simulink model "StateMachinaTesting"  (R2016a)
settings: Solver=VariableStepAuto  StartTime=0.0  StopTime=orbit_length*40  RelTol=1e-3
values from neighbouring files (symbols this model uses):
  A = eye(16,16)    [full_input_list.m]
  B = zeros(16,1)    [full_input_list.m]
  C = blkdiag(eye(3,3),zeros(3,3),eye(10,10))    [full_input_list.m]
  counter = 0    [full_input_list.m]
  deltaT = 0.00001    (= 1e-05)    [full_input_list.m]
  H = C    [full_input_list.m]
  kd = 0.5    [full_input_list.m]    (also in initACS.m = 0.01)
  kp = 1    [full_input_list.m]    (also in initACS.m = 0.01)
  OpModes = [0 0 0]    [full_input_list.m]
  OpTimes = [0 1 2]    [full_input_list.m]
  Q_k = zeros(16,16)    [full_input_list.m]
  R = R_k    [full_input_list.m]
  SeperationTime = 30000    [full_input_list.m]
  sim_start_time = (JD - JD_GPS0) * 24*60*60 - UTC_leap_seconds_wrt_GPS    (= 36000.0287935)    [full_input_list.m]
  st = 1/freq    (= 0.0125)    [full_input_list.m]    (also in initSimulink.m)
  u_k = zeros(16,1)    [full_input_list.m]
  w_k = zeros(16,1)    [full_input_list.m]
  x0 = [0 ... (first row only)    [full_input_list.m]
  Z_k = zeros(16,1)    [full_input_list.m]
undefined symbols (not defined in the file or in its folder): DiscIntNeverNeededParam, Earth, G_igrf, gyro_DCM_BS, H_igrf, I_undeployed, IAU, km, Kschmidt, mag_variance, n, R_mean, sat2, WGS84
libraries: simulink x29, dspmathops x24, aerolibutil x20, aerolibtransform2 x20, vrlib x15, aerolibgravity2 x5, dspinverses x4, SimMainLibrary x3, dspmtrx3 x1, lib_violet_env x1
(part 1 of 4)
settings Model: Creator=npp26  LastModifiedBy=gtc59

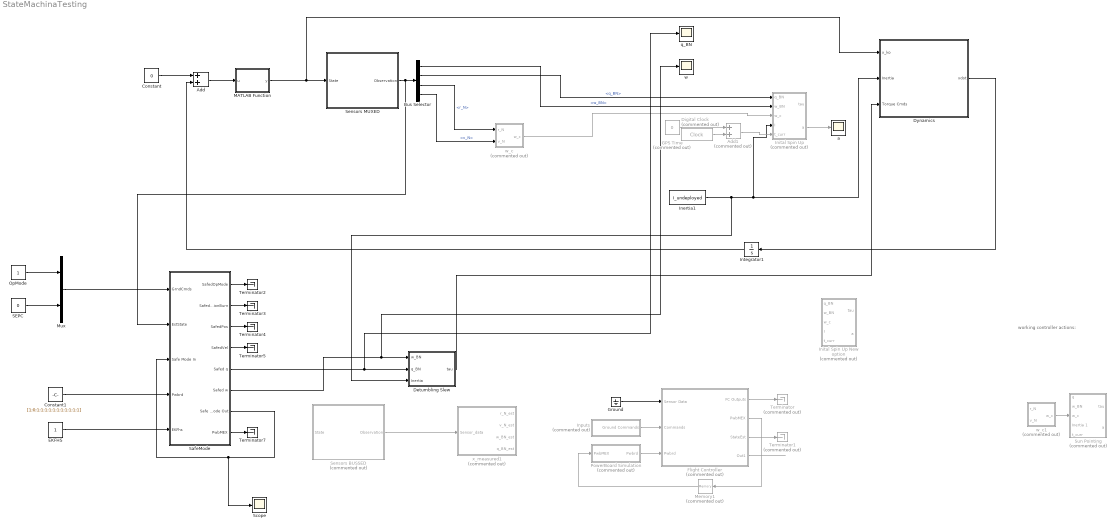
== system StateMachinaTesting ==
  note: working controller actions:
  Add : Sum
  Add1 : Sum  Commented=on
  Bus Selector : BusSelector  OutputSignals=w_BN,q_BN,r_N,v_N
  Constant : Constant  Value=0
  Constant1 : Constant  Value=[1;0;1;1;1;1;1;1;1;1;1;1;1]
  Detumbling Slew : Subsystem  TreatAsAtomicUnit=on
  Digital Clock : DigitalClock  Commented=on
  "Dynamics " : Subsystem
  EKFHS : Constant
  Flight Controller : Subsystem  Commented=on
  GPS Time : Constant  Commented=on  Value=0
  Ground : Ground
  Inertia1 : Constant  Value=I_undeployed
  Inital Spin Up : Subsystem  Commented=on  TreatAsAtomicUnit=on
  Inital Spin Up New option : Subsystem  Commented=on  TreatAsAtomicUnit=on
  Inputs : Subsystem  Commented=on
  Integrator1 : Integrator  InitialCondition=x0
  MATLAB Function : MATLAB Function  TreatAsAtomicUnit=on
  Memory1 : Memory  Commented=on  InheritSampleTime=on
  Mux : Mux  Inputs=2
  OpMode : Constant
  PowerBoard Simulation : Subsystem  Commented=on
  SEPC : Constant  Value=0
  SafeMode : Subsystem
  Scope : Scope
  Sensors BUSSED : Subsystem  Commented=on
  Sensors MUXED : Subsystem
  Sun Pointing : Subsystem  Commented=on  TreatAsAtomicUnit=on
  Terminator : Terminator  Commented=on
  Terminator1 : Terminator  Commented=on
  Terminator{2..5,7} (5 alike) : Terminator
  a : Scope
  q_BN : Scope
  w : Scope
  w_c : Subsystem  Commented=on
  w_c1 : Subsystem  Commented=on
  x_measured1 : Subsystem  Commented=on
  wires:
  "Dynamics "/1("xdot  ") -> Integrator1/1
  Constant/1 -> Add/1
  Integrator1/1 -> Add/2
  Add/1 -> MATLAB Function/1(u)
  Inertia1/1 -> Detumbling Slew/3("Inertia "), Inital Spin Up/4("I "), "Dynamics "/2(Inertia)
  Inputs/1(Ground Commands) -> Flight Controller/2(Commands)
  PowerBoard Simulation/1(Pwbrd) -> Flight Controller/3(Pwbrd)
  Flight Controller/2(PwbMEX) -> Memory1/1
  Memory1/1 -> PowerBoard Simulation/1(PwbMEX)
  Ground/1 -> Flight Controller/1(Sensor Data)
  Flight Controller/1(FC Outputs) -> Terminator/1
  Flight Controller/3(StateEst) -> Terminator1/1
  Flight Controller/4(Out1) -> ?
  Bus Selector/2 -> Inital Spin Up/1(q_BN)  "<q_BN>"
  Bus Selector/1 -> Inital Spin Up/2(w_BN)  "<w_BN>"
  Sensors BUSSED/1(Observation) -> x_measured1/1(Sensor_data)
  Sensors MUXED/1(Observation) -> SafeMode/2(EstState), Bus Selector/1
  MATLAB Function/1(y) -> Sensors MUXED/1(State), "Dynamics "/1("x_ko ")
  Bus Selector/3 -> w_c/1(r_N)  "<r_N>"
  Bus Selector/4 -> w_c/2(v_N)  "<v_N>"
  w_c/1(w_c) -> Inital Spin Up/3(w_c)
  Inital Spin Up/2(a) -> a/1
  w_c1/1(w_c) -> Sun Pointing/3(w_c)
  GPS Time/1 -> Add1/1
  Digital Clock/1 -> Add1/2
  Add1/1 -> Inital Spin Up/5(t_curr)
  SafeMode/5(Safed q) -> q_BN/1, Detumbling Slew/2(q_BN)
  SafeMode/6(Safed w) -> w/1, Detumbling Slew/1(w_BN)
  SafeMode/1(SafedOpMode) -> Terminator2/1
  SafeMode/2(SafedSeperationBurn) -> Terminator3/1
  SafeMode/3(SafedPos) -> Terminator4/1
  SafeMode/4(SafedVel) -> Terminator5/1
  SafeMode/7(Safe Mode Out) -> Scope/1, SafeMode/3(Safe Mode In)
  SafeMode/8(PwbMEX) -> Terminator7/1
  OpMode/1 -> Mux/1
  SEPC/1 -> Mux/2
  Mux/1 -> SafeMode/1(GrndCmds)
  Constant1/1 -> SafeMode/4(Pwbrd)
  EKFHS/1 -> SafeMode/5("EKFhs ")
  Detumbling Slew/1(tau) -> "Dynamics "/3(Torque Cmds)

== system StateMachinaTesting/Detumbling Slew ==
  note: Regulator
      | - q_target = [0 0 0 1]
      | - w_target = [0 0 0]
  note: Markley Regulator
      | This regulator takes the current directional quaterion vector, the target quaterion, the intertial matrix, and the current angular velocity to determine the required torque necessary to the slew.
      |
      | The equation is 7.8 listed on page 290 of Fundamentals of Spacecraft Attitude Determination and Control. The input I is currently not defined. Also important to the equation is equation 7.2
  w_BN : Inport
  q_BN : Inport  Port=2
  "Inertia " : Inport  Port=3
  3x3 Cross Product : aerolibutil/3x3 Cross Product
  Add : Sum  Inputs=+++
  Constant : Constant  Commented=on  Value=[0;0;0]
  Gain : Gain  Gain=-1
  Gain1 : Gain  Gain=kp
  Gain2 : Gain  Gain=-1
  Gain3 : Gain  Gain=kd
  Gain4 : Gain  Gain=-1
  Product : Product  Multiplication=Matrix(*)
  Quaternion Inverse : aerolibutil/Quaternion Inverse
  Quaternion Multiplication : aerolibutil/Quaternion Multiplication
  Selector : Selector  InputPortWidth=4  IndexOptions=Index vector (dialog)  Indices=[1 2 3]  OutputSizes=1
  Target q : Constant  Value=[ 0 0 0 1 ]
  tau : Outport
  wires:
  Target q/1 -> Quaternion Inverse/1
  Quaternion Multiplication/1 -> Selector/1
  Selector/1 -> Gain1/1
  Gain1/1 -> Gain/1
  Gain3/1 -> Gain2/1
  w_BN/1 -> 3x3 Cross Product/1, Gain3/1, Product/2
  Gain/1 -> Add/1
  Gain2/1 -> Add/2
  "Inertia "/1 -> Product/1
  Product/1 -> 3x3 Cross Product/2
  3x3 Cross Product/1 -> Gain4/1
  Gain4/1 -> Add/3
  Add/1 -> tau/1
  Quaternion Inverse/1 -> Quaternion Multiplication/1
  q_BN/1 -> Quaternion Multiplication/2

== system StateMachinaTesting/Dynamics  ==
  note: State x {16x1} =
      | x y z - Position
      | xdot ydot zdot - Velocity
      | xddot yddot zddot - Accel
      | w1 w2 w3 - Angular Vel
      | q1 q2 q3 q4 - Quaternion
  "x_ko " : Inport
  Inertia : Inport  Port=2
  Torque Cmds : Inport  Port=3
  Dynamics of the System : MATLAB Function  TreatAsAtomicUnit=on
  "xdot  " : Outport
  wires:
  Dynamics of the System/1(xdot) -> "xdot  "/1
  Torque Cmds/1 -> Dynamics of the System/3(torques)
  Inertia/1 -> Dynamics of the System/2(Inertia)
  "x_ko "/1 -> Dynamics of the System/1(x_ko)

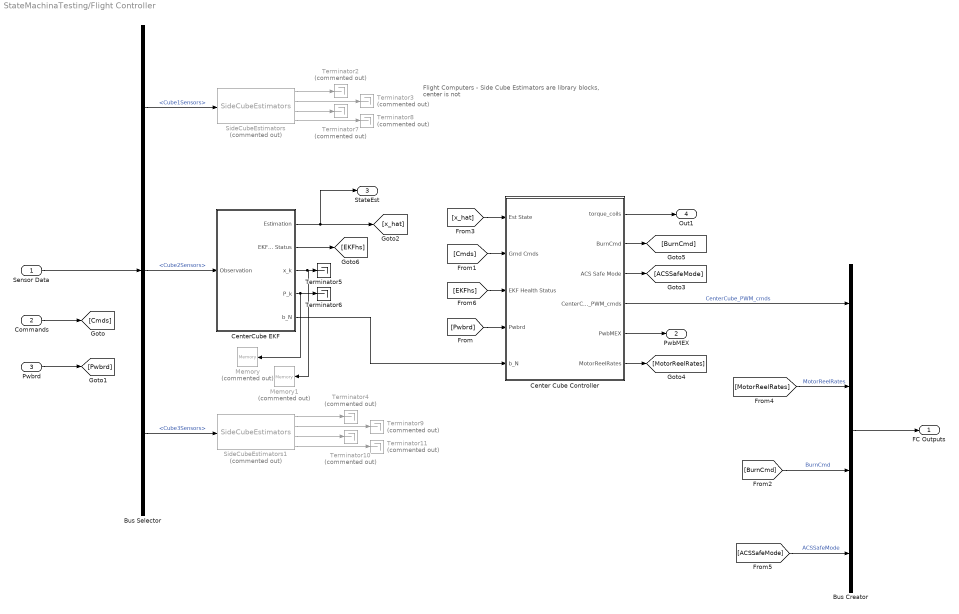
== system StateMachinaTesting/Flight Controller ==
  note: Flight Computers
      | - Side Cube Estimators are library blocks, center is not
  Sensor Data : Inport
  Commands : Inport  Port=2
  Pwbrd : Inport  Port=3
  Bus Creator : BusCreator  Inputs=4
  Bus Selector : BusSelector  OutputSignals=Cube1Sensors,Cube2Sensors,Cube3Sensors
  Center Cube Controller : Subsystem
  CenterCube EKF : Subsystem
  Memory : Memory  Commented=on
  Memory1 : Memory  Commented=on
  SideCubeEstimators : SimMainLibrary/SideCubeEstimators  Commented=on
  SideCubeEstimators1 : SimMainLibrary/SideCubeEstimators  Commented=on
  Terminator{2..4,7..11} (8 alike) : Terminator  Commented=on
  Terminator5 : Terminator
  Terminator6 : Terminator
  FC Outputs : Outport
  PwbMEX : Outport  Port=2
  StateEst : Outport  Port=3
  Out1 : Outport  Port=4
  wires:
  Sensor Data/1 -> Bus Selector/1
  Bus Selector/1 -> SideCubeEstimators/1  "<Cube1Sensors>"
  Bus Selector/2 -> CenterCube EKF/1(Observation)  "<Cube2Sensors>"
  Bus Selector/3 -> SideCubeEstimators1/1  "<Cube3Sensors>"
  SideCubeEstimators/1 -> Terminator2/1
  Bus Creator/1 -> FC Outputs/1
  Commands/1 -> [Cmds]
  [Cmds] -> Center Cube Controller/2(Grnd Cmds)
  Center Cube Controller/3(ACS Safe Mode) -> [ACSSafeMode]
  Center Cube Controller/2(BurnCmd) -> [BurnCmd]
  [BurnCmd] -> Bus Creator/3  "BurnCmd"
  CenterCube EKF/2(EKF Health Status) -> [EKFhs]
  [EKFhs] -> Center Cube Controller/3("EKF Health Status ")
  Pwbrd/1 -> [Pwbrd]
  [Pwbrd] -> Center Cube Controller/4(Pwbrd)
  Center Cube Controller/5(PwbMEX) -> PwbMEX/1
  CenterCube EKF/1(Estimation) -> [x_hat], StateEst/1
  [x_hat] -> Center Cube Controller/1(Est State)
  Center Cube Controller/4(CenterCube_PWM_cmds) -> Bus Creator/1  "CenterCube_PWM_cmds"
  SideCubeEstimators/2 -> Terminator3/1
  CenterCube EKF/3(x_k) -> Memory1/1, Terminator5/1
  CenterCube EKF/4(P_k) -> Terminator6/1, Memory/1
  SideCubeEstimators/3 -> Terminator7/1
  SideCubeEstimators/4 -> Terminator8/1
  SideCubeEstimators1/1 -> Terminator4/1
  SideCubeEstimators1/2 -> Terminator9/1
  SideCubeEstimators1/3 -> Terminator10/1
  SideCubeEstimators1/4 -> Terminator11/1
  [ACSSafeMode] -> Bus Creator/4  "ACSSafeMode"
  Center Cube Controller/6(MotorReelRates) -> [MotorReelRates]
  [MotorReelRates] -> Bus Creator/2  "MotorReelRates"
  Center Cube Controller/1(torque_coils) -> Out1/1
  CenterCube EKF/5(b_N) -> Center Cube Controller/5(b_N)

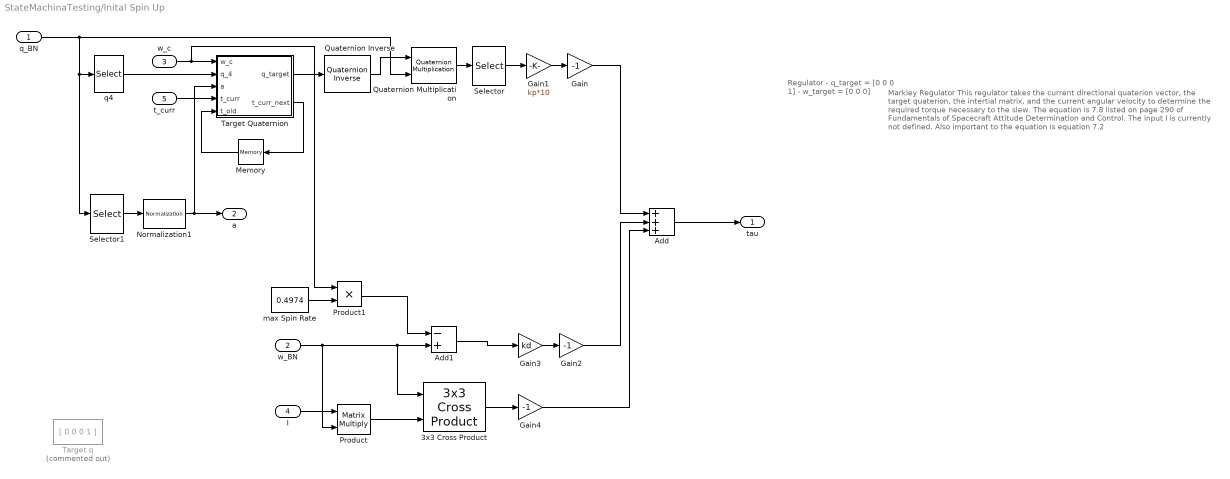
== system StateMachinaTesting/Inital Spin Up ==
  note: Regulator
      | - q_target = [0 0 0 1]
      | - w_target = [0 0 0]
  note: Markley Regulator
      | This regulator takes the current directional quaterion vector, the target quaterion, the intertial matrix, and the current angular velocity to determine the required torque necessary to the slew.
      |
      | The equation is 7.8 listed on page 290 of Fundamentals of Spacecraft Attitude Determination and Control. The input I is currently not defined. Also important to the equation is equation 7.2
  q_BN : Inport
  w_BN : Inport  Port=2
  w_c : Inport  Port=3
  "I " : Inport  Port=4
  t_curr : Inport  Port=5
  3x3 Cross Product : aerolibutil/3x3 Cross Product
  Add : Sum  Inputs=+++
  Add1 : Sum  Inputs=-+
  Gain : Gain  Gain=-1
  Gain1 : Gain  Gain=kp*10
  Gain2 : Gain  Gain=-1
  Gain3 : Gain  Gain=kd
  Gain4 : Gain  Gain=-1
  Memory : Memory
  Normalization1 : dspmathops/Normalization  NormType=2-norm  Bias=1e-10  NormOver=Each column  Dimension=1  outputDataTypeStr=Inherit: Same as product output  outputLastDataTypeStr=Inherit: Same as product output  outputMin=[]  outputMax=[]  accumDataTypeStr=Inherit: Same as product output  accumLastDataTypeStr=Inherit: Same as product output  roundingMode=Floor  overflowMode=off
  Product : Product  Multiplication=Matrix(*)
  Product1 : Product
  Quaternion Inverse : aerolibutil/Quaternion Inverse
  Quaternion Multiplication : aerolibutil/Quaternion Multiplication
  Selector : Selector  InputPortWidth=4  IndexOptions=Index vector (dialog)  Indices=[1 2 3]  OutputSizes=1
  Selector1 : Selector  InputPortWidth=4  IndexOptions=Index vector (dialog)  Indices=[1 2 3]  OutputSizes=1
  Target Quaternion : Subsystem
  Target q : Constant  Commented=on  Value=[ 0 0 0 1 ]
  max Spin Rate : Constant  Value=0.4974
  q4 : Selector  InputPortWidth=4  IndexOptions=Index vector (dialog)  Indices=[4]  OutputSizes=1
  tau : Outport
  a : Outport  Port=2
  wires:
  Target Quaternion/1(q_target) -> Quaternion Inverse/1
  Quaternion Multiplication/1 -> Selector/1
  Selector/1 -> Gain1/1
  Gain1/1 -> Gain/1
  Gain3/1 -> Gain2/1
  w_BN/1 -> Product/2, Add1/2, 3x3 Cross Product/1
  Add/1 -> tau/1
  Gain/1 -> Add/1
  Gain2/1 -> Add/2
  "I "/1 -> Product/1
  Product/1 -> 3x3 Cross Product/2
  3x3 Cross Product/1 -> Gain4/1
  Gain4/1 -> Add/3
  w_c/1 -> Product1/1, Target Quaternion/1(w_c)
  Selector1/1 -> Normalization1/1
  Normalization1/1 -> a/1, Target Quaternion/3(a)
  t_curr/1 -> Target Quaternion/4(t_curr)
  q4/1 -> Target Quaternion/2(q_4)
  Target Quaternion/2(t_curr_next) -> Memory/1
  Memory/1 -> Target Quaternion/5(t_old)
  q_BN/1 -> Quaternion Multiplication/2, Selector1/1, q4/1
  max Spin Rate/1 -> Product1/2
  Add1/1 -> Gain3/1
  Product1/1 -> Add1/1
  Quaternion Inverse/1 -> Quaternion Multiplication/1

== system StateMachinaTesting/Inital Spin Up New option ==
  note: Markley Regulator
      | This regulator takes the current directional quaterion vector, the target quaterion, the intertial matrix, and the current angular velocity to determine the required torque necessary to the slew.
      |
      | The equation is 7.8 listed on page 290 of Fundamentals of Spacecraft Attitude Determination and Control. The input I is currently not defined. Also important to the equation is equation 7.2
  note: Regulator
      | - q_target = [0 0 0 1]
      | - w_target = [0 0 0]
  q_BN : Inport
  w_BN : Inport  Port=2
  w_c : Inport  Port=3
  "I " : Inport  Port=4
  t_curr : Inport  Port=5
  3x3 Cross Product : aerolibutil/3x3 Cross Product
  Add : Sum  Inputs=+++
  Add1 : Sum  Inputs=-+
  Add2 : Sum  Inputs=-+
  Gain : Gain  Gain=-1
  Gain1 : Gain  Gain=kp
  Gain2 : Gain  Gain=-1
  Gain3 : Gain  Gain=kd
  Gain4 : Gain  Gain=-1
  Normalization1 : dspmathops/Normalization  NormType=2-norm  Bias=1e-10  NormOver=Each column  Dimension=1  outputDataTypeStr=Inherit: Same as product output  outputLastDataTypeStr=Inherit: Same as product output  outputMin=[]  outputMax=[]  accumDataTypeStr=Inherit: Same as product output  accumLastDataTypeStr=Inherit: Same as product output  roundingMode=Floor  overflowMode=off
  Product : Product  Multiplication=Matrix(*)
  Product1 : Product
  Selector1 : Selector  InputPortWidth=4  IndexOptions=Index vector (dialog)  Indices=[1 2 3]  OutputSizes=1
  Terminator : Terminator
  max Spin Rate : Constant  Value=0.4974
  tau : Outport
  a : Outport  Port=2
  wires:
  Normalization1/1 -> a/1
  Selector1/1 -> Normalization1/1
  Gain4/1 -> Add/3
  3x3 Cross Product/1 -> Gain4/1
  Product/1 -> Add1/1, 3x3 Cross Product/2
  "I "/1 -> Product/1
  Gain2/1 -> Add/2
  Gain/1 -> Add/1
  Add/1 -> tau/1
  w_BN/1 -> 3x3 Cross Product/1, Add2/2, Product/2
  Gain3/1 -> Gain2/1
  Gain1/1 -> Gain/1
  Add1/1 -> Gain1/1
  q_BN/1 -> Selector1/1
  t_curr/1 -> Terminator/1
  w_c/1 -> Add1/2, Product1/1
  max Spin Rate/1 -> Product1/2
  Product1/1 -> Add2/1
  Add2/1 -> Gain3/1

== system StateMachinaTesting/Inputs ==
  Bus Creator : BusCreator  Inputs=2
  Choose Mode : MATLAB Function  TreatAsAtomicUnit=on
  Clock : Clock
  Constant : Constant  Value=OpModes
  Constant1 : Constant  Value=OpTimes
  Constant2 : Constant  Value=SeperationTime
  Ground Commands : Outport
  wires:
  Constant/1 -> Choose Mode/3(OpModes)
  Constant1/1 -> Choose Mode/2(OpTimes)
  Clock/1 -> Choose Mode/1(time)
  Constant2/1 -> Choose Mode/4(SeperationTime)
  Choose Mode/1(OM) -> Bus Creator/1  "OpMode"
  Choose Mode/2(SEPC) -> Bus Creator/2  "SeperationCommand"
  Bus Creator/1 -> Ground Commands/1

== system StateMachinaTesting/PowerBoard Simulation ==
  PwbMEX : Inport
  Bus Creator : BusCreator  Inputs=2
  Bus Creator1 : BusCreator  Inputs=8
  Bus Creator2 : BusCreator  Inputs=3
  Bus Creator3 : BusCreator  Inputs=2
  Bus Creator4 : BusCreator  Inputs=2
  Choose Mode : MATLAB Function  TreatAsAtomicUnit=on
  Clock : Clock
  Constant : Constant  Value=OpModes
  Constant1 : Constant  Value=OpTimes
  Constant2 : Constant  Value=SeperationTime
  Sensor Ak Signals : Subsystem
  Torquer Shunts : Subsystem
  Pwbrd : Outport
  wires:
  Constant/1 -> Choose Mode/4(OpModes)
  Constant1/1 -> Choose Mode/3(OpTimes)
  Clock/1 -> Choose Mode/2(time)
  Constant2/1 -> Choose Mode/5(SeperationTime)
  Choose Mode/1(OM) -> Bus Creator/1  "PbOpMode"
  Choose Mode/2(SEPC) -> Bus Creator/2  "PbSepCmmd"
  Bus Creator/1 -> Bus Creator4/1  "PwbrdCmmds"
  Sensor Ak Signals/4(Out4) -> Bus Creator1/4  "Accel2Ak"
  Sensor Ak Signals/3(Out3) -> Bus Creator1/3  "Accel1Ak"
  Sensor Ak Signals/1(Out1) -> Bus Creator1/1  "Mag1Ak"
  Sensor Ak Signals/2(Out2) -> Bus Creator1/2  "Mag2Ak"
  Bus Creator1/1 -> Bus Creator3/1  "SensorsAk"
  Torquer Shunts/1(Torquer X1 Shunt) -> Bus Creator2/1  "TC_X1"
  Torquer Shunts/2(Torquer Y1 Shunt) -> Bus Creator2/2  "TC_Y1"
  Torquer Shunts/3(Torquer Z1 Shunt) -> Bus Creator2/3  "TC_Z1"
  Bus Creator2/1 -> Bus Creator3/2  "TorquerAk"
  Bus Creator3/1 -> Bus Creator4/2  "ADCSAks"
  Bus Creator4/1 -> Pwbrd/1
  Sensor Ak Signals/5(Out5) -> Bus Creator1/5  "Gyro1Ak"
  Sensor Ak Signals/6(Out6) -> Bus Creator1/6  "Gyro2Ak"
  Sensor Ak Signals/7(Out7) -> Bus Creator1/7  "SunS1Ak"
  Sensor Ak Signals/8(Out8) -> Bus Creator1/8  "SunS2Ak"
  PwbMEX/1 -> Choose Mode/1(PwbMEX)

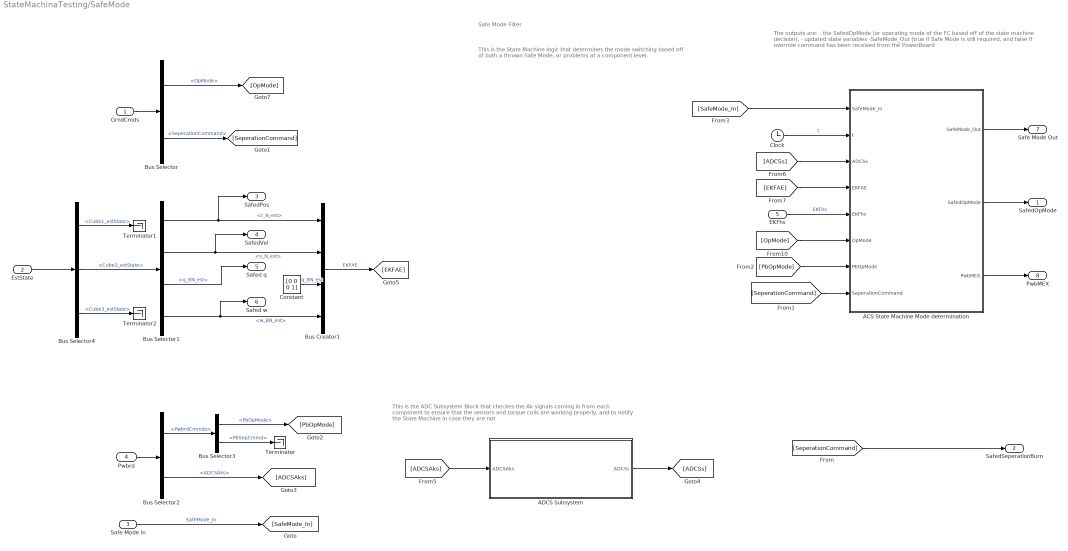
== system StateMachinaTesting/SafeMode ==
  note: This is the State Machine logic that determines the mode switching based off of both a thrown Safe Mode, or problems at a component level.
  note: Safe Mode Filter
  note: The outputs are:
      | - the SafedOpMode (or operating mode of the FC based off of the state machine decision),
      | - updated state variables
      | -SafeMode_Out (true if Safe Mode is still required, and false if override command has been received from the PowerBoard
  note: This is the ADC Subsystem Block that checkes the Ak signals coming in from each component to ensure that the sensors and torque coils are working properly, and to notify the State Machine in case they are not
  GrndCmds : Inport
  EstState : Inport  Port=2
  Safe Mode In : Inport  Port=3
  Pwbrd : Inport  Port=4
  "EKFhs " : Inport  Port=5
  ACS State Machine Mode determination : MATLAB Function  TreatAsAtomicUnit=on
  ADCS Subsystem : Subsystem
  Bus Creator1 : BusCreator  Inputs='r_N_est','v_N_est','q_BN_est','w_BN_est'
  Bus Selector : BusSelector  OutputSignals=OpMode,SeperationCommand
  Bus Selector1 : BusSelector  OutputSignals=r_N_est,v_N_est,q_BN_est,w_BN_est
  Bus Selector2 : BusSelector  OutputSignals=PwbrdCmmds,ADCSAks
  Bus Selector3 : BusSelector  OutputSignals=PbOpMode,PbSepCmmd
  Bus Selector4 : BusSelector  OutputSignals=Cube1_estState,Cube2_estState,Cube3_estState
  Clock : Clock
  Constant : Constant  Value=[0 0 0 1]
  Terminator : Terminator
  Terminator1 : Terminator
  Terminator2 : Terminator
  SafedOpMode : Outport
  SafedSeperationBurn : Outport  Port=2
  SafedPos : Outport  Port=3
  SafedVel : Outport  Port=4
  Safed q : Outport  Port=5
  Safed w : Outport  Port=6
  Safe Mode Out : Outport  Port=7
  PwbMEX : Outport  Port=8
  wires:
  Clock/1 -> ACS State Machine Mode determination/2(t)  "t"
  "EKFhs "/1 -> ACS State Machine Mode determination/5(EKFhs)  "EKFhs"
  [ADCSs] -> ACS State Machine Mode determination/3(ADCSs)
  Bus Selector1/4 -> Safed w/1, Bus Creator1/4  "<w_BN_est>"
  Bus Selector1/3 -> Safed q/1  "<q_BN_est>"
  Bus Selector1/2 -> SafedVel/1, Bus Creator1/2  "<v_N_est>"
  Bus Selector1/1 -> SafedPos/1, Bus Creator1/1  "<r_N_est>"
  EstState/1 -> Bus Selector4/1
  Bus Selector/1 -> [OpMode]  "<OpMode>"
  GrndCmds/1 -> Bus Selector/1
  Safe Mode In/1 -> [SafeMode_In]  "SafeMode_In"
  ACS State Machine Mode determination/1(SafeMode_Out) -> Safe Mode Out/1
  Bus Selector/2 -> [SeperationCommand]  "<SeperationCommand>"
  [SeperationCommand] -> SafedSeperationBurn/1
  [SeperationCommand] -> ACS State Machine Mode determination/8(SeperationCommand)
  Pwbrd/1 -> Bus Selector2/1
  Bus Selector2/2 -> [ADCSAks]  "<ADCSAks>"
  [ADCSAks] -> ADCS Subsystem/1("ADCSAks ")
  Bus Selector2/1 -> Bus Selector3/1  "<PwbrdCmmds>"
  Bus Selector3/1 -> [PbOpMode]  "<PbOpMode>"
  [OpMode] -> ACS State Machine Mode determination/6(OpMode)
  [PbOpMode] -> ACS State Machine Mode determination/7(PbOpMode)
  Bus Creator1/1 -> [EKFAE]  "EKFAE"
  [EKFAE] -> ACS State Machine Mode determination/4(EKFAE)
  ACS State Machine Mode determination/2(SafedOpMode) -> SafedOpMode/1
  ACS State Machine Mode determination/3(PwbMEX) -> PwbMEX/1
  Bus Selector3/2 -> Terminator/1  "<PbSepCmmd>"
  ADCS Subsystem/1("ADCSs ") -> [ADCSs]
  [SafeMode_In] -> ACS State Machine Mode determination/1(SafeMode_In)
  Constant/1 -> Bus Creator1/3  "q_BN_est"
  Bus Selector4/2 -> Bus Selector1/1  "<Cube2_estState>"
  Bus Selector4/1 -> Terminator1/1  "<Cube1_estState>"
  Bus Selector4/3 -> Terminator2/1  "<Cube3_estState>"

== system StateMachinaTesting/Sensors BUSSED ==
  note: Sensor Blocks:
      | -The SideCube blocks are library blocks to because they are the same
      | -Center Cube is not
  State : Inport
  Bus Creator1 : BusCreator  Inputs=3
  Bus Selector1 : BusSelector  OutputSignals=Cube1State,Cube2State,Cube3State
  Center Cube Sensors : Subsystem
  Mux to Bus conversion : Subsystem
  SideCubeSensors : Subsystem  AncestorBlock=SimMainLibrary/SideCubeSensors
  SideCubeSensors1 : Subsystem  AncestorBlock=SimMainLibrary/SideCubeSensors
  Observation : Outport
  wires:
  Bus Creator1/1 -> Observation/1
  Bus Selector1/1 -> SideCubeSensors/1(State)  "<Cube1State>"
  SideCubeSensors/1(Sensors) -> Bus Creator1/1  "Cube1Sensors"
  SideCubeSensors1/1(Sensors) -> Bus Creator1/3  "Cube3Sensors"
  Center Cube Sensors/1(Sensors) -> Bus Creator1/2  "Cube2Sensors"
  Bus Selector1/2 -> Center Cube Sensors/1(State)  "<Cube2State>"
  Bus Selector1/3 -> SideCubeSensors1/1(State)  "<Cube3State>"
  State/1 -> Mux to Bus conversion/1(In1)
  Mux to Bus conversion/1(Out1) -> Bus Selector1/1

== system StateMachinaTesting/Sensors MUXED ==
  note: Sensor Blocks:
      | -The SideCube blocks are library blocks to because they are the same
      | -Center Cube is not
  State : Inport
  Bus Creator4 : BusCreator  Inputs=4
  Center Cube Sensors : Subsystem  Commented=on
  Demux : Demux  Outputs=16
  Mux{,1..3} (4 alike) : Mux  Inputs=3
  Mux4 : Mux
  Scope : Scope
  Terminator2 : Terminator
  Observation : Outport
  wires:
  State/1 -> Demux/1
  Demux/2 -> Mux/2
  Demux/1 -> Mux/1
  Demux/3 -> Mux/3
  Demux/5 -> Mux1/2
  Demux/6 -> Mux1/3
  Demux/4 -> Mux1/1
  Mux/1 -> Scope/1, Bus Creator4/1  "r_N"
  Mux1/1 -> Bus Creator4/2  "v_N"
  Demux/8 -> Mux2/2
  Demux/9 -> Mux2/3
  Demux/7 -> Mux2/1
  Mux2/1 -> Terminator2/1  "xddot"
  Demux/12 -> Mux3/3
  Demux/11 -> Mux3/2
  Demux/10 -> Mux3/1
  Mux3/1 -> Bus Creator4/4  "w_BN"
  Demux/13 -> Mux4/1
  Demux/14 -> Mux4/2
  Demux/15 -> Mux4/3
  Demux/16 -> Mux4/4
  Mux4/1 -> Bus Creator4/3  "q_BN"
  Bus Creator4/1 -> Observation/1

== system StateMachinaTesting/Sun Pointing ==
  note: Regulator
      | - q_target = [0 0 1 0]
      | - w_target = [0 0 0]
  q : Inport
  w_BN : Inport  Port=2
  w_c : Inport  Port=3
  Inertia 1 : Inport  Port=4
  t_curr : Inport  Port=5
  3x3 Cross Product : aerolibutil/3x3 Cross Product
  Add4 : Sum  Inputs=+++
  Gain : Gain  Gain=-1
  Gain1 : Gain  Gain=kp
  Gain4 : Gain  Gain=-1
  Gain5 : Gain  Gain=kd
  Gain6 : Gain  Gain=-1
  Normalization1 : dspmathops/Normalization  NormType=2-norm  Bias=1e-10  NormOver=Each column  Dimension=1  outputDataTypeStr=Inherit: Same as product output  outputLastDataTypeStr=Inherit: Same as product output  outputMin=[]  outputMax=[]  accumDataTypeStr=Inherit: Same as product output  accumLastDataTypeStr=Inherit: Same as product output  roundingMode=Floor  overflowMode=off
  Product4 : Product  Multiplication=Matrix(*)
  Quaternion Inverse1 : aerolibutil/Quaternion Inverse
  Quaternion Multiplication1 : aerolibutil/Quaternion Multiplication
  Selector1 : Selector  InputPortWidth=4  IndexOptions=Index vector (dialog)  Indices=[1 2 3]  OutputSizes=1
  Selector2 : Selector  InputPortWidth=4  IndexOptions=Index vector (dialog)  Indices=[1 2 3]  OutputSizes=1
  Target Quaternion : Subsystem
  Terminator : Terminator
  q4 : Selector  InputPortWidth=4  IndexOptions=Index vector (dialog)  Indices=[4]  OutputSizes=1
  tau : Outport
  a : Outport  Port=2
  wires:
  q/1 -> Quaternion Multiplication1/2, Selector1/1, q4/1
  Quaternion Multiplication1/1 -> Selector2/1
  Selector2/1 -> Gain1/1
  Gain1/1 -> Gain/1
  Gain5/1 -> Gain4/1
  w_BN/1 -> 3x3 Cross Product/1, Gain5/1, Product4/2
  Gain/1 -> Add4/1
  Gain4/1 -> Add4/2
  Inertia 1/1 -> Product4/1
  Product4/1 -> 3x3 Cross Product/2
  3x3 Cross Product/1 -> Gain6/1
  Gain6/1 -> Add4/3
  Add4/1 -> tau/1
  w_c/1 -> Target Quaternion/1(w_c)
  q4/1 -> Target Quaternion/2(q4)
  Target Quaternion/1(q_target) -> Quaternion Inverse1/1
  Selector1/1 -> Normalization1/1
  Normalization1/1 -> a/1
  t_curr/1 -> Terminator/1
  Quaternion Inverse1/1 -> Quaternion Multiplication1/1

== system StateMachinaTesting/w_c ==
  r_N : Inport
  v_N : Inport  Port=2
  Cross Product : vrlib/Utilities/Cross Product
  Normalization1 : dspmathops/Normalization  NormType=2-norm  Bias=1e-10  NormOver=Each column  Dimension=1  outputDataTypeStr=Inherit: Same as product output  outputLastDataTypeStr=Inherit: Same as product output  outputMin=[]  outputMax=[]  accumDataTypeStr=Inherit: Same as product output  accumLastDataTypeStr=Inherit: Same as product output  roundingMode=Floor  overflowMode=off
  Scope : Scope
  w_c : Outport
  wires:
  Cross Product/1 -> Normalization1/1
  r_N/1 -> Cross Product/1
  v_N/1 -> Cross Product/2
  Normalization1/1 -> w_c/1, Scope/1

== system StateMachinaTesting/w_c1 ==
  r_N : Inport
  v_N : Inport  Port=2
  Cross Product : vrlib/Utilities/Cross Product
  Normalization1 : dspmathops/Normalization  NormType=2-norm  Bias=1e-10  NormOver=Each column  Dimension=1  outputDataTypeStr=Inherit: Same as product output  outputLastDataTypeStr=Inherit: Same as product output  outputMin=[]  outputMax=[]  accumDataTypeStr=Inherit: Same as product output  accumLastDataTypeStr=Inherit: Same as product output  roundingMode=Floor  overflowMode=off
  Scope : Scope
  w_c : Outport
  wires:
  Cross Product/1 -> Normalization1/1
  r_N/1 -> Cross Product/1
  v_N/1 -> Cross Product/2
  Normalization1/1 -> w_c/1, Scope/1

== system StateMachinaTesting/x_measured1 ==
  Sensor_data : Inport
  Bus Selector1 : BusSelector  OutputSignals=Cube2Sensors.accelerometer_1,Cube2Sensors.w_BN_1,Cube2Sensors.sun_B,Cube2Sensors.r_N,Cube2Sensors.magnetometer_1,Cube2Sensors.time
  Lookup Tables : Subsystem
  Name change : MATLAB Function  TreatAsAtomicUnit=on
  Name change1 : MATLAB Function  TreatAsAtomicUnit=on
  Terminator : Terminator
  Terminator1 : Terminator
  q_N from Sensors : Subsystem
  vis viva : MATLAB Function  TreatAsAtomicUnit=on
  r_N_est : Outport
  v_N_est : Outport  Port=2
  w_BN_est : Outport  Port=3
  q_BN_est : Outport  Port=4
  wires:
  Bus Selector1/6 -> Lookup Tables/2(time)  "<time>"
  Bus Selector1/2 -> q_N from Sensors/1(B_B)  "<w_BN_1>"
  q_N from Sensors/1(q_N) -> q_BN_est/1  "q_BN_est"
  Sensor_data/1 -> Bus Selector1/1
  q_N from Sensors/2(Q) -> Terminator/1
  Lookup Tables/1(B_N) -> q_N from Sensors/3(B_N)
  Bus Selector1/3 -> q_N from Sensors/2(V_sun_B)  "<sun_B>"
  Lookup Tables/2(V_sun_N) -> q_N from Sensors/4(V_sun_N)
  Bus Selector1/4 -> Name change/1(u), Lookup Tables/1(x_pos)  "<r_N>"
  Name change1/1(y) -> w_BN_est/1  "w_BN_est"
  Bus Selector1/1 -> Name change1/1(u)  "<accelerometer_1>"
  Bus Selector1/5 -> Terminator1/1  "<magnetometer_1>"
  Name change/1(y) -> r_N_est/1, vis viva/1(x)  "r_N_est"
  vis viva/1(xdot) -> v_N_est/1  "v_N_est"

== system StateMachinaTesting/Flight Controller/Center Cube Controller ==
  note: Why does torque coils suddenly become PWM?
  Est State : Inport
  Grnd Cmds : Inport  Port=2
  "EKF Health Status " : Inport  Port=3
  Pwbrd : Inport  Port=4
  b_N : Inport  Port=5
  Attitude Compensator : Subsystem
  Memory : Memory  InheritSampleTime=on
  Motor Control Placeholder : Subsystem
  SafeMode : Subsystem
  Terminator1 : Terminator
  Terminator2 : Terminator
  Terminator3 : Terminator
  Torque Coil Management : Subsystem
  torque_coils : Outport
  BurnCmd : Outport  Port=2
  ACS Safe Mode : Outport  Port=3
  CenterCube_PWM_cmds : Outport  Port=4
  PwbMEX : Outport  Port=5
  MotorReelRates : Outport  Port=6
  wires:
  Memory/1 -> SafeMode/3(Safe Mode In)
  Attitude Compensator/2(SepBurn) -> BurnCmd/1, Torque Coil Management/1(BurnCmd)
  SafeMode/2(SafedSeperationBurn) -> Attitude Compensator/2(SafedSepBurn)
  SafeMode/3(SafedPos) -> Terminator3/1
  SafeMode/4(SafedVel) -> Terminator2/1
  Est State/1 -> SafeMode/2(EstState)
  SafeMode/1(SafedOpMode) -> Attitude Compensator/1(SafedOpMode), Motor Control Placeholder/2(SafedOpMode)
  Grnd Cmds/1 -> SafeMode/1(GrndCmds)
  "EKF Health Status "/1 -> SafeMode/5("EKFhs ")
  Pwbrd/1 -> SafeMode/4(Pwbrd)
  Torque Coil Management/2(torque_coils) -> torque_coils/1
  Torque Coil Management/1(CenterCube_PWM_cmds) -> CenterCube_PWM_cmds/1
  Attitude Compensator/3(Tau1) -> Torque Coil Management/4(tau_B)
  SafeMode/5(Safed q) -> Torque Coil Management/2(q_BN), Attitude Compensator/3(q2)
  SafeMode/7(Safe Mode Out) -> Memory/1, ACS Safe Mode/1
  SafeMode/8(PwbMEX) -> PwbMEX/1
  SafeMode/6(Safed w) -> Motor Control Placeholder/1(spin rate), Torque Coil Management/3(w), Attitude Compensator/4(w2)
  Attitude Compensator/1(OpMode) -> Terminator1/1
  Motor Control Placeholder/1(motor cmd) -> MotorReelRates/1
  b_N/1 -> Torque Coil Management/5(b_N)

== system StateMachinaTesting/Flight Controller/CenterCube EKF ==
  note: The output of this block should be both an estimate of the attitude based off of the sensor data (as well as historical values), as well as a boolean value for the EKF Health Status determined by the covariance matrix.
  note: Placeholder
  note: This is the Kalman filter. The goal of the Kalman filter is to obtain an estimate of the craft's attitude based off of sensor data from the previous state. it does so by taking in sensor data, creating an estimate of the attitude from said data, saving it, and comparing the next state iteration with its estimate in order to determine the accuracy and the validity of each component of the sensor data.
  note: L/E Kalman Filter
  note: State x {16x1} =
      | x y z - Position
      | xdot ydot zdot - Velocity
      | xddot yddot zddot - Accel
      | w1 w2 w3 - Angular Vel
      | q1 q2 q3 q4 - Quaternion
  Observation : Inport
  Add2 : Sum  Commented=on  Inputs=+-
  Bus Creator : BusCreator  Inputs=4
  Bus Creator1 : BusCreator  Inputs=3
  Bus Creator2 : BusCreator  Inputs=4
  Bus Creator3 : BusCreator  Inputs=4
  Constant1 : Constant
  H2 : Constant  Commented=on  Value=H
  Identity Matrix : dspmtrx3/Identity Matrix  Commented=on  Inherit=off  N=16  Ts=1  dataType=double  isSigned=on  wordLen=16  udDataType=sfix(16)  fracBitsMode=Best precision  numFracBits=15  OutDataTypeStr=double  LastOutDataTypeStr=double
  Kalman Gain and Estamated State Computation : Subsystem  Commented=on
  "New State Prediction " : Subsystem  Commented=on
  Observation1 : InportShadow
  P_previous : Constant  Commented=on
  Product2 : Product  Commented=on  Multiplication=Matrix(*)
  Product7 : Product  Commented=on  Multiplication=Matrix(*)
  Y computation : Subsystem  Commented=on
  state_previous : Constant  Commented=on
  x_measured : Subsystem
  x_measured1 : Subsystem
  Estimation : Outport
  EKF Health Status : Outport  Port=2
  x_k : Outport  Port=3
  P_k : Outport  Port=4
  b_N : Outport  Port=5
  wires:
  x_measured1/2(v_N_est) -> Bus Creator3/2, Bus Creator2/2, Bus Creator/2  "v_N_est"
  Observation/1 -> x_measured1/1(Sensor_data)
  Bus Creator/1 -> Bus Creator1/2  "Cube2_estState"
  x_measured1/4(q_BN_est) -> Bus Creator3/3, Bus Creator2/3, Bus Creator/3  "q_BN_est"
  x_measured1/1(r_N_est) -> Bus Creator3/1, Bus Creator2/1, Bus Creator/1  "r_N_est"
  x_measured1/3(w_BN_est) -> Bus Creator3/4, Bus Creator2/4, Bus Creator/4  "w_BN_est"
  Bus Creator1/1 -> Estimation/1
  Bus Creator2/1 -> Bus Creator1/1  "Cube1_estState"
  Bus Creator3/1 -> Bus Creator1/3  "Cube3_estState"
  Constant1/1 -> EKF Health Status/1
  P_previous/1 -> "New State Prediction "/1(P_k-1)
  state_previous/1 -> "New State Prediction "/2(x_k-1)
  "New State Prediction "/1(P_kp) -> Product7/2, Kalman Gain and Estamated State Computation/1(P_kp)
  Kalman Gain and Estamated State Computation/2(x_k) -> x_k/1
  Identity Matrix/1 -> Add2/1
  H2/1 -> Product2/2
  Product2/1 -> Add2/2
  Add2/1 -> Product7/1
  Product7/1 -> P_k/1
  Kalman Gain and Estamated State Computation/1(K) -> Product2/1
  "New State Prediction "/2("x_kp  ") -> Kalman Gain and Estamated State Computation/2(x_kp)
  Y computation/1(Y) -> Kalman Gain and Estamated State Computation/3(Y)
  x_measured/1(x_measured) -> Y computation/1(In1)
  x_measured/2(B_N) -> b_N/1
  Observation1/1 -> x_measured/1(Sensor_data)

== system StateMachinaTesting/Inital Spin Up/Target Quaternion ==
  w_c : Inport
  q_4 : Inport  Port=2
  a : Inport  Port=3
  t_curr : Inport  Port=4
  t_old : Inport  Port=5
  Abs : Abs
  Add1 : Sum  Inputs=+-
  Aligned : Subsystem  TreatAsAtomicUnit=on
  Aligned1 : Subsystem  TreatAsAtomicUnit=on
  Demux : Demux  Outputs=3
  If : If  NumInputs=4  IfExpression=(u1 <= u4) & (u2 <= u4) & (u3 <=u4)
  Not Aligned : Subsystem  Commented=on  TreatAsAtomicUnit=on
  Phi_new : Merge
  Product : Product
  Scope : Scope
  Scope1 : Scope
  Trigonometric Function1 : Trigonometry
  Trigonometric Function2 : Trigonometry  Operator=cos
  Unary Minus : UnaryMinus
  Vector Concatenate : Concatenate
  tolerance : Constant  Value=1e-3
  q_target : Outport
  t_curr_next : Outport  Port=2
  wires:
  Vector Concatenate/1 -> Scope1/1, q_target/1
  w_c/1 -> Product/1, Add1/1
  Product/1 -> Vector Concatenate/1
  Trigonometric Function1/1 -> Product/2
  Trigonometric Function2/1 -> Vector Concatenate/2
  Phi_new/1 -> Trigonometric Function2/1, Trigonometric Function1/1
  Demux/1 -> If/1
  Demux/2 -> If/2
  Demux/3 -> If/3
  t_curr/1 -> t_curr_next/1, Aligned1/2(t_curr), Aligned/2(t_curr)
  q_4/1 -> Aligned1/1(q4), Aligned/1(q4)
  Aligned1/1(Phi/2_new) -> Phi_new/2
  Aligned/1(Phi/2_new) -> Phi_new/1
  If/1 -> Aligned/Action
  If/2 -> Aligned1/Action
  tolerance/1 -> If/4
  Add1/1 -> Abs/1
  Abs/1 -> Scope/1, Demux/1
  a/1 -> Unary Minus/1
  Unary Minus/1 -> Add1/2
  t_old/1 -> Aligned1/3(t_old), Aligned/3(t_old)

== system StateMachinaTesting/PowerBoard Simulation/Sensor Ak Signals ==
  Acc1 : Constant
  Acc2 : Constant
  Gyro1 : Constant
  Gyro2 : Constant
  Mag1 : Constant
  Mag2 : Constant
  SunSensor1 : Constant
  SunSensor2 : Constant
  Out1 : Outport
  Out2 : Outport  Port=2
  Out3 : Outport  Port=3
  Out4 : Outport  Port=4
  Out5 : Outport  Port=5
  Out6 : Outport  Port=6
  Out7 : Outport  Port=7
  Out8 : Outport  Port=8
  wires:
  Acc2/1 -> Out4/1
  Acc1/1 -> Out3/1
  Mag2/1 -> Out2/1
  Mag1/1 -> Out1/1
  Gyro2/1 -> Out6/1
  Gyro1/1 -> Out5/1
  SunSensor1/1 -> Out7/1
  SunSensor2/1 -> Out8/1

== system StateMachinaTesting/PowerBoard Simulation/Torquer Shunts ==
  Constant : Constant
  Constant2 : Constant
  Constant4 : Constant
  Torquer X1 Shunt : Outport
  Torquer Y1 Shunt : Outport  Port=2
  Torquer Z1 Shunt : Outport  Port=3
  wires:
  Constant4/1 -> Torquer Z1 Shunt/1
  Constant2/1 -> Torquer Y1 Shunt/1
  Constant/1 -> Torquer X1 Shunt/1

== system StateMachinaTesting/SafeMode/ADCS Subsystem ==
  "ADCSAks " : Inport
  Bus Selector : BusSelector  OutputSignals=SensorsAk,TorquerAk
  Bus Selector1 : BusSelector  OutputSignals=Mag1Ak,Mag2Ak,Accel1Ak,Accel2Ak,Gyro1Ak,Gyro2Ak,SunS1Ak,SunS2Ak
  Bus Selector2 : BusSelector  OutputSignals=TC_X1,TC_Y1,TC_Z1
  Data Type Conversion : DataTypeConversion
  IMU : Subsystem
  Logical Operator1 : Logic  Operator=OR  AllPortsSameDT=off  OutDataTypeStr=boolean
  Magnetic Torquers : Subsystem
  Mux : Mux
  Mux1 : Mux  Inputs=3
  Mux3 : Mux  Inputs=3
  Mux4 : Mux  Inputs=2
  Mux5 : Mux  Inputs=2
  "ADCSs " : Outport
  wires:
  Bus Selector2/3 -> Magnetic Torquers/3(Magnetometer Z1)  "<TC_Z1>"
  Bus Selector2/2 -> Magnetic Torquers/2(Magnetometer Y1)  "<TC_Y1>"
  Mux1/1 -> "ADCSs "/1  "ADCS Health"
  Mux4/1 -> Mux1/2  "ADCS Sectional Status"
  IMU/1(Magnetometer) -> Mux/1  "Magnetometer Health"
  IMU/3(Accelerometer) -> Mux/3  "Accelerometer Health"
  IMU/2("Gyro ") -> Mux/2  "Gyro Health"
  IMU/5(IMU Health) -> Mux4/1, Logical Operator1/1  "IMU Health"
  Magnetic Torquers/2("Y Torquer Status ") -> Mux3/2  "Y Torquer Status"
  Magnetic Torquers/1(X Torquer Status) -> Mux3/1  "X Torquer Status"
  Bus Selector2/1 -> Magnetic Torquers/1(Magnetorquer X1)  "<TC_X1>"
  IMU/4("Sun Sensor ") -> Mux/4  "Sun Sensor"
  Logical Operator1/1 -> Mux1/1  "ADCS Functional Status"
  Mux5/1 -> Mux1/3  "ADCS Component Status"
  Mux3/1 -> Data Type Conversion/1  "Torquer Status Array"
  Magnetic Torquers/4(Actuator Health) -> Mux4/2, Logical Operator1/2  "Actuator Health"
  Mux/1 -> Mux5/1  "Sensor Status Array"
  Magnetic Torquers/3(Z Torquer Status) -> Mux3/3  "Z Torquer Status"
  "ADCSAks "/1 -> Bus Selector/1
  Bus Selector/2 -> Bus Selector2/1  "<TorquerAk>"
  Bus Selector/1 -> Bus Selector1/1  "<SensorsAk>"
  Bus Selector1/1 -> IMU/1(Magnetometer 1)  "<Mag1Ak>"
  Bus Selector1/2 -> IMU/2(Magnetometer 2)  "<Mag2Ak>"
  Bus Selector1/3 -> IMU/3(Accelerometer 1)  "<Accel1Ak>"
  Bus Selector1/4 -> IMU/4(" Accelerometer 2")  "<Accel2Ak>"
  Bus Selector1/5 -> IMU/5(Gyro 1)  "<Gyro1Ak>"
  Bus Selector1/6 -> IMU/6(Gyro 2)  "<Gyro2Ak>"
  Bus Selector1/7 -> IMU/7(Sun Sensor 1)  "<SunS1Ak>"
  Bus Selector1/8 -> IMU/8(Sun Sensor 2)  "<SunS2Ak>"
  Data Type Conversion/1 -> Mux5/2

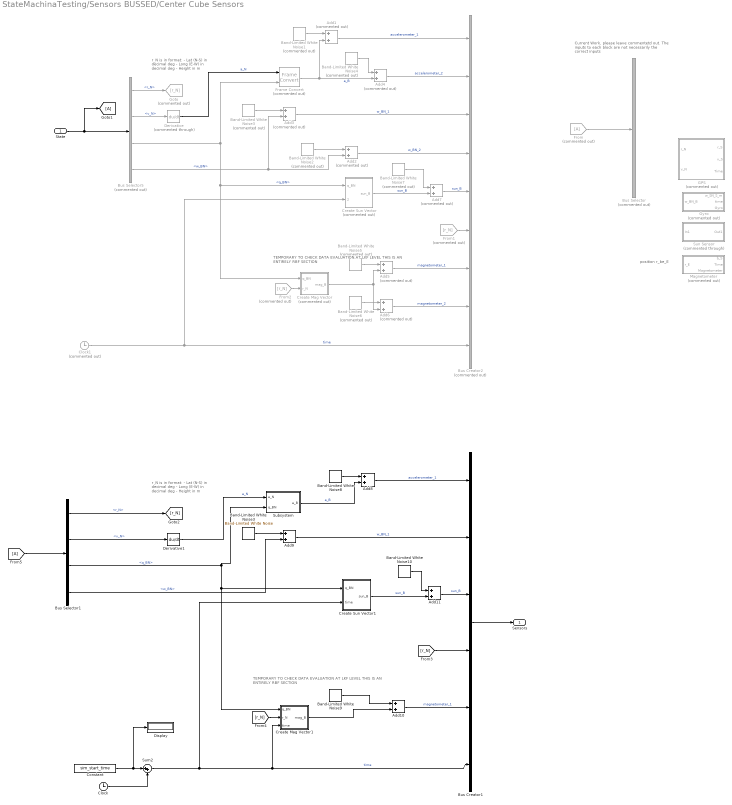
== system StateMachinaTesting/Sensors BUSSED/Center Cube Sensors ==
  note: position r_be_E
  note: Current Work, please leave commentetd out.
      | The inputs to each block are not necessarily
      | the correct inputs
  note: TEMPORARY TO CHECK DATA EVALUATION AT LKF LEVEL
      | THIS IS AN ENTIRELY RBF SECTION
  note: r_N is in format:
      | - Lat (N-S) in decimal deg
      | - Long (E-W) in decimal deg
      | - Height in m
  note: TEMPORARY TO CHECK DATA EVALUATION AT LKF LEVEL
      | THIS IS AN ENTIRELY RBF SECTION
  note: r_N is in format:
      | - Lat (N-S) in decimal deg
      | - Long (E-W) in decimal deg
      | - Height in m
  State : Inport
  Add{1..7} (7 alike) : Sum  Commented=on
  Add{8..11} (4 alike) : Sum
  Band-Limited White  Noise3 : simulink/Sources/Band-Limited White Noise  Cov=[1e-5]  Ts=0.1  seed=[23341]
  Band-Limited White Noise1 : simulink/Sources/Band-Limited White Noise  Commented=on  Cov=[0.1]  Ts=st  seed=[23341]
  Band-Limited White Noise10 : simulink/Sources/Band-Limited White Noise  Cov=[0.1]  Ts=0.1  seed=[23341]
  Band-Limited White Noise{2..3,5..7} (5 alike) : simulink/Sources/Band-Limited White Noise  Commented=on  Cov=[0.1]  Ts=0.1  seed=[23341]
  Band-Limited White Noise4 : simulink/Sources/Band-Limited White Noise  Commented=on  Cov=[0.1]  Ts=st  seed=[23341]
  Band-Limited White Noise8 : simulink/Sources/Band-Limited White Noise  Cov=[0.1]  Ts=st  seed=[23341]
  Band-Limited White Noise9 : simulink/Sources/Band-Limited White Noise  Cov=[0.1]  Ts=0.1  seed=[23341]
  Bus Creator1 : BusCreator  Inputs=6
  Bus Creator2 : BusCreator  Commented=on  Inputs=9
  Bus Selector : BusSelector  Commented=on  OutputSignals=r_N,v_N,q_BN,w_BN
  Bus Selector1 : BusSelector  OutputSignals=r_N,v_N,q_BN,w_BN
  Bus Selector5 : BusSelector  Commented=on  OutputSignals=r_N,v_N,q_BN,w_BN
  Clock : Clock
  Clock1 : Clock  Commented=on
  Constant : Constant  Value=sim_start_time
  Create Mag Vector : Subsystem  Commented=on
  Create Mag Vector1 : Subsystem
  Create Sun Vector : Subsystem  Commented=on  AncestorBlock=SimMainLibrary/SideCubeSensors/Create Sun Vector
  Create Sun Vector1 : Subsystem  AncestorBlock=SimMainLibrary/SideCubeSensors/Create Sun Vector
  Derivative : Derivative  Commented=through
  Derivative1 : Derivative
  Display : Display
  Frame Convert : SimMainLibrary/SideCubeSensors/Frame Convert  Commented=on
  From : From  Commented=on
  From1 : From  Commented=on  GotoTag=r_N
  From2 : From  Commented=on  GotoTag=r_N
  GPS : Subsystem  Commented=on
  Goto : Goto  Commented=on  GotoTag=r_N
  Gyro : Subsystem  Commented=on
  Magnetometer : Subsystem  Commented=on
  Subsystem : Subsystem
  Sum2 : Sum  Inputs=|++
  Sun Sensor : Subsystem  Commented=through
  Sensors : Outport
  wires:
  Bus Selector5/1 -> Goto/1  "<r_N>"
  Add1/1 -> Bus Creator2/1  "accelerometer_1"
  Bus Selector5/2 -> Derivative/1  "<v_N>"
  Band-Limited White Noise1/1 -> Add1/1
  Frame Convert/1 -> Add4/2, Add1/2  "a_B"
  Add4/1 -> Bus Creator2/2  "accelerometer_2"
  Band-Limited White Noise2/1 -> Add2/1
  Band-Limited White Noise3/1 -> Add3/1
  Bus Selector5/4 -> Add3/2, Add2/2  "<w_BN>"
  State/1 -> [A], Bus Selector5/1
  Band-Limited White Noise4/1 -> Add4/1
  Derivative/1 -> Frame Convert/1  "a_N"
  Add7/1 -> Bus Creator2/5  "sun_B"
  Clock1/1 -> Create Sun Vector/2(GPS time), Bus Creator2/9  "time"
  Add2/1 -> Bus Creator2/4  "w_BN_2"
  Add3/1 -> Bus Creator2/3  "w_BN_1"
  Band-Limited White Noise7/1 -> Add7/1
  Create Sun Vector/1(sun_B) -> Add7/2  "sun_B"
  From1/1 -> Bus Creator2/6
  Add6/1 -> Bus Creator2/8  "magnetometer_2"
  Create Mag Vector/1(mag_B) -> Add6/2, Add5/2
  Band-Limited White Noise6/1 -> Add6/1
  Add5/1 -> Bus Creator2/7  "magnetometer_1"
  Bus Selector5/3 -> Create Mag Vector/1(q_BN), Create Sun Vector/1(q_BN), Frame Convert/2  "<q_BN>"
  Band-Limited White Noise5/1 -> Add5/1
  From2/1 -> Create Mag Vector/2(r_N)
  From/1 -> Bus Selector/1
  Add8/1 -> Bus Creator1/1  "accelerometer_1"
  Band-Limited White Noise8/1 -> Add8/1
  Subsystem/1(a_B) -> Add8/2  "a_B"
  Band-Limited White  Noise3/1 -> Add9/1
  [A] -> Bus Selector1/1
  Bus Creator1/1 -> Sensors/1
  Derivative1/1 -> Subsystem/1("a_N ")  "a_N"
  Add11/1 -> Bus Creator1/3  "sun_B"
  Sum2/1 -> Create Sun Vector1/2(time), Create Mag Vector1/3(time), Bus Creator1/6  "time"
  Add9/1 -> Bus Creator1/2  "w_BN_1"
  Band-Limited White Noise10/1 -> Add11/1
  Create Sun Vector1/1(sun_B) -> Add11/2  "sun_B"
  [r_N] -> Bus Creator1/4
  Create Mag Vector1/1(mag_B) -> Add10/2
  Add10/1 -> Bus Creator1/5  "magnetometer_1"
  Band-Limited White Noise9/1 -> Add10/1
  [r_N] -> Create Mag Vector1/2(r_N)
  Bus Selector1/1 -> [r_N]  "<r_N>"
  Bus Selector1/2 -> Derivative1/1  "<v_N>"
  Bus Selector1/3 -> Subsystem/2(q_BN), Create Mag Vector1/1(q_BN), Create Sun Vector1/1(q_BN)  "<q_BN>"
  Bus Selector1/4 -> Add9/2  "<w_BN>"
  Constant/1 -> Sum2/1, Display/1
  Clock/1 -> Sum2/2

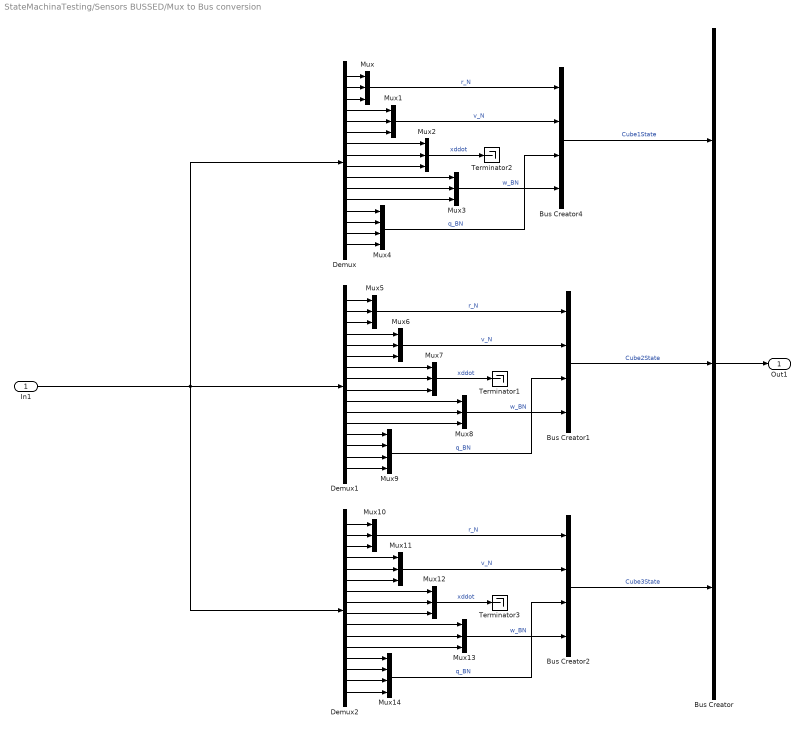
== system StateMachinaTesting/Sensors BUSSED/Mux to Bus conversion ==
  In1 : Inport
  Bus Creator : BusCreator  Inputs=3
  Bus Creator1 : BusCreator  Inputs=4
  Bus Creator2 : BusCreator  Inputs=4
  Bus Creator4 : BusCreator  Inputs=4
  Demux : Demux  Outputs=16
  Demux1 : Demux  Outputs=16
  Demux2 : Demux  Outputs=16
  Mux{,1..3,5..8,10..13} (12 alike) : Mux  Inputs=3
  Mux14 : Mux
  Mux4 : Mux
  Mux9 : Mux
  Terminator1 : Terminator
  Terminator2 : Terminator
  Terminator3 : Terminator
  Out1 : Outport
  wires:
  Mux4/1 -> Bus Creator4/3  "q_BN"
  Demux/11 -> Mux3/2
  Demux/12 -> Mux3/3
  Demux/8 -> Mux2/2
  Demux/6 -> Mux1/3
  Bus Creator4/1 -> Bus Creator/1  "Cube1State"
  Demux/16 -> Mux4/4
  Demux/4 -> Mux1/1
  Demux/10 -> Mux3/1
  Mux3/1 -> Bus Creator4/4  "w_BN"
  Demux/13 -> Mux4/1
  Demux/14 -> Mux4/2
  Mux2/1 -> Terminator2/1  "xddot"
  Mux/1 -> Bus Creator4/1  "r_N"
  Demux/2 -> Mux/2
  Demux/3 -> Mux/3
  Demux/1 -> Mux/1
  Demux/15 -> Mux4/3
  Mux1/1 -> Bus Creator4/2  "v_N"
  Demux/5 -> Mux1/2
  Demux/7 -> Mux2/1
  Demux/9 -> Mux2/3
  Mux9/1 -> Bus Creator1/3  "q_BN"
  Demux1/11 -> Mux8/2
  Demux1/12 -> Mux8/3
  Demux1/8 -> Mux7/2
  Demux1/6 -> Mux6/3
  Bus Creator1/1 -> Bus Creator/2  "Cube2State"
  Demux1/16 -> Mux9/4
  Demux1/4 -> Mux6/1
  Demux1/10 -> Mux8/1
  Mux8/1 -> Bus Creator1/4  "w_BN"
  Demux1/13 -> Mux9/1
  Demux1/14 -> Mux9/2
  Mux7/1 -> Terminator1/1  "xddot"
  Mux5/1 -> Bus Creator1/1  "r_N"
  Demux1/2 -> Mux5/2
  Demux1/3 -> Mux5/3
  Demux1/1 -> Mux5/1
  Demux1/15 -> Mux9/3
  Mux6/1 -> Bus Creator1/2  "v_N"
  Demux1/5 -> Mux6/2
  Demux1/7 -> Mux7/1
  Demux1/9 -> Mux7/3
  Mux14/1 -> Bus Creator2/3  "q_BN"
  In1/1 -> Demux2/1, Demux1/1, Demux/1
  Demux2/11 -> Mux13/2
  Demux2/12 -> Mux13/3
  Demux2/8 -> Mux12/2
  Demux2/6 -> Mux11/3
  Bus Creator2/1 -> Bus Creator/3  "Cube3State"
  Demux2/16 -> Mux14/4
  Demux2/4 -> Mux11/1
  Demux2/10 -> Mux13/1
  Mux13/1 -> Bus Creator2/4  "w_BN"
  Demux2/13 -> Mux14/1
  Demux2/14 -> Mux14/2
  Mux12/1 -> Terminator3/1  "xddot"
  Mux10/1 -> Bus Creator2/1  "r_N"
  Demux2/2 -> Mux10/2
  Demux2/3 -> Mux10/3
  Demux2/1 -> Mux10/1
  Demux2/15 -> Mux14/3
  Mux11/1 -> Bus Creator2/2  "v_N"
  Demux2/5 -> Mux11/2
  Demux2/7 -> Mux12/1
  Demux2/9 -> Mux12/3
  Bus Creator/1 -> Out1/1

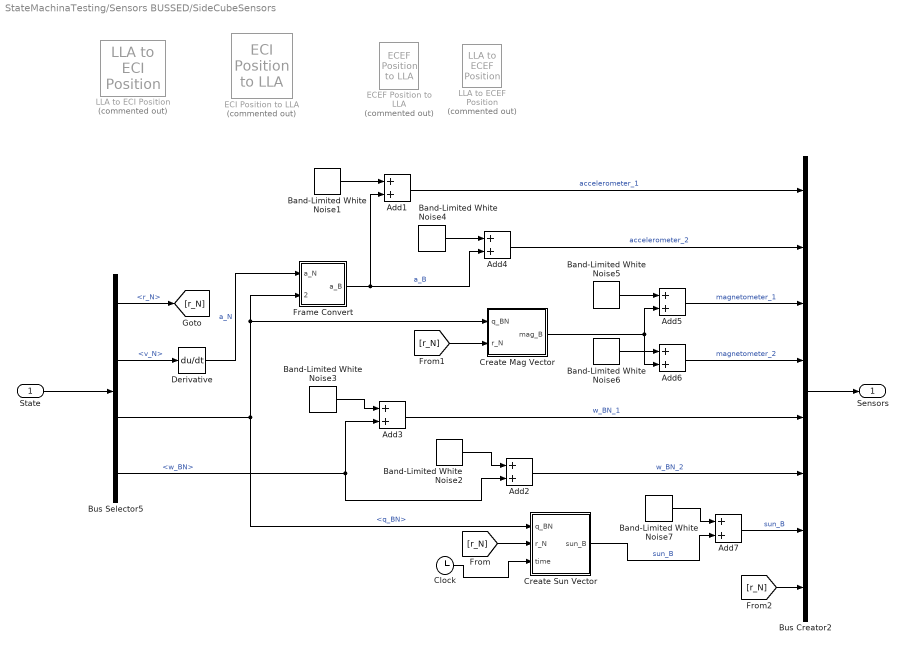
== system StateMachinaTesting/Sensors BUSSED/SideCubeSensors ==
  State : Inport
  Add{1..7} (7 alike) : Sum
  Band-Limited White Noise{1..7} (7 alike) : simulink/Sources/Band-Limited White Noise  Cov=[0.1]  Ts=0.1  seed=[23341]
  Bus Creator2 : BusCreator  Inputs=8
  Bus Selector5 : BusSelector  OutputSignals=r_N,v_N,q_BN,w_BN
  Clock : Clock
  Create Mag Vector : Subsystem
  Create Sun Vector : Subsystem
  Derivative : Derivative
  ECEF Position to LLA : aerolibtransform2/ECEF Position to LLA  Commented=on  units=Metric (MKS)  ptype=Earth (WGS84)  F=1/298.257223563  R=6378137
  ECI Position to LLA : aerolibtransform2/ECI Position to LLA  Commented=on  red=IAU-2000/2006  year=2016  month=September  day=20  hour=0  min=0  sec=0  deltaT=Sec  errorflag=Error  extraparamflag=off  eunits=Metric (MKS)  earthmodel=WGS84  flat=1/298.257223563  eqradius=6378137
      settings: AttributesFormatString=%<red>
  Frame Convert : Subsystem
  LLA to ECEF Position : aerolibtransform2/LLA to ECEF Position  Commented=on  units=Metric (MKS)  ptype=Earth (WGS84)  F=1/298.257223563  R=6378137
  LLA to ECI Position : aerolibtransform2/LLA to ECI Position  Commented=on  red=IAU-2000/2006  year=2013  month=January  day=1  hour=0  min=0  sec=0  deltaT=Day  errorflag=Error  extraparamflag=on  eunits=Metric (MKS)  earthmodel=WGS84  flat=1/298.257223563  eqradius=6378137
      settings: AttributesFormatString=%<red>
  Sensors : Outport
  wires:
  Create Sun Vector/1(sun_B) -> Add7/2  "sun_B"
  Band-Limited White Noise7/1 -> Add7/1
  Add3/1 -> Bus Creator2/5  "w_BN_1"
  Add2/1 -> Bus Creator2/6  "w_BN_2"
  Clock/1 -> Create Sun Vector/3(time)
  Add7/1 -> Bus Creator2/7  "sun_B"
  Add6/1 -> Bus Creator2/4  "magnetometer_2"
  Create Mag Vector/1(mag_B) -> Add5/2, Add6/2
  Band-Limited White Noise6/1 -> Add6/1
  Band-Limited White Noise5/1 -> Add5/1
  [r_N] -> Create Mag Vector/2(r_N)
  Add5/1 -> Bus Creator2/3  "magnetometer_1"
  [r_N] -> Create Sun Vector/2(r_N)
  Derivative/1 -> Frame Convert/1(a_N)  "a_N"
  Band-Limited White Noise4/1 -> Add4/1
  Bus Creator2/1 -> Sensors/1
  State/1 -> Bus Selector5/1
  Bus Selector5/4 -> Add3/2, Add2/2  "<w_BN>"
  Band-Limited White Noise3/1 -> Add3/1
  Bus Selector5/3 -> Frame Convert/2(q_BN), Create Mag Vector/1(q_BN), Create Sun Vector/1(q_BN)  "<q_BN>"
  Band-Limited White Noise2/1 -> Add2/1
  Add4/1 -> Bus Creator2/2  "accelerometer_2"
  Frame Convert/1(a_B) -> Add1/2, Add4/2  "a_B"
  Band-Limited White Noise1/1 -> Add1/1
  Bus Selector5/2 -> Derivative/1  "<v_N>"
  Add1/1 -> Bus Creator2/1  "accelerometer_1"
  Bus Selector5/1 -> [r_N]  "<r_N>"
  [r_N] -> Bus Creator2/8

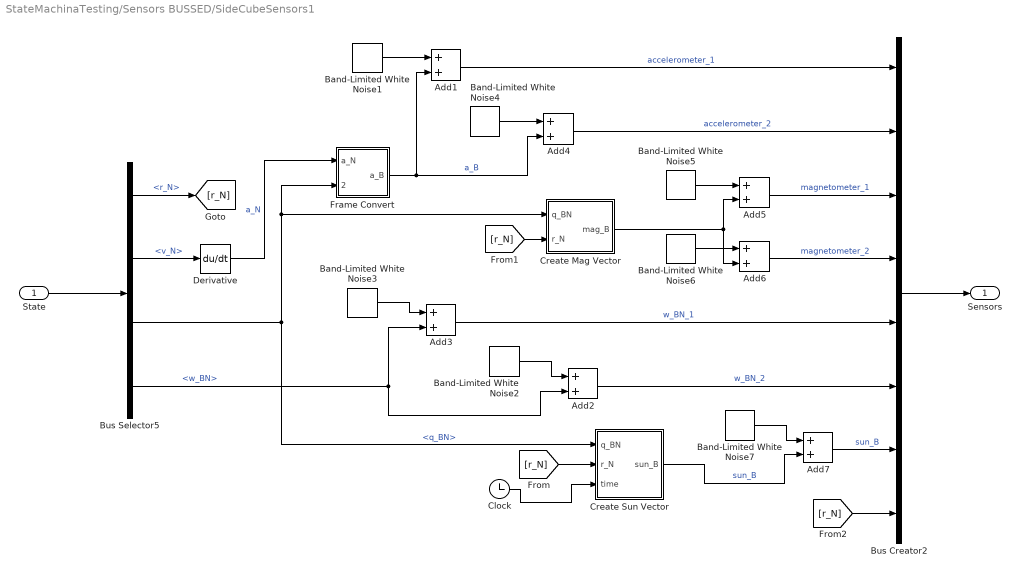
== system StateMachinaTesting/Sensors BUSSED/SideCubeSensors1 ==
  State : Inport
  Add{1..7} (7 alike) : Sum
  Band-Limited White Noise{1..7} (7 alike) : simulink/Sources/Band-Limited White Noise  Cov=[0.1]  Ts=0.1  seed=[23341]
  Bus Creator2 : BusCreator  Inputs=8
  Bus Selector5 : BusSelector  OutputSignals=r_N,v_N,q_BN,w_BN
  Clock : Clock
  Create Mag Vector : Subsystem
  Create Sun Vector : Subsystem
  Derivative : Derivative
  Frame Convert : Subsystem
  Sensors : Outport
  wires:
  Create Sun Vector/1(sun_B) -> Add7/2  "sun_B"
  Band-Limited White Noise7/1 -> Add7/1
  Add3/1 -> Bus Creator2/5  "w_BN_1"
  Add2/1 -> Bus Creator2/6  "w_BN_2"
  Clock/1 -> Create Sun Vector/3(time)
  Add7/1 -> Bus Creator2/7  "sun_B"
  Add6/1 -> Bus Creator2/4  "magnetometer_2"
  Create Mag Vector/1(mag_B) -> Add5/2, Add6/2
  Band-Limited White Noise6/1 -> Add6/1
  Band-Limited White Noise5/1 -> Add5/1
  [r_N] -> Create Mag Vector/2(r_N)
  Add5/1 -> Bus Creator2/3  "magnetometer_1"
  [r_N] -> Create Sun Vector/2(r_N)
  Derivative/1 -> Frame Convert/1(a_N)  "a_N"
  Band-Limited White Noise4/1 -> Add4/1
  Bus Creator2/1 -> Sensors/1
  State/1 -> Bus Selector5/1
  Bus Selector5/4 -> Add3/2, Add2/2  "<w_BN>"
  Band-Limited White Noise3/1 -> Add3/1
  Bus Selector5/3 -> Frame Convert/2(q_BN), Create Mag Vector/1(q_BN), Create Sun Vector/1(q_BN)  "<q_BN>"
  Band-Limited White Noise2/1 -> Add2/1
  Add4/1 -> Bus Creator2/2  "accelerometer_2"
  Frame Convert/1(a_B) -> Add1/2, Add4/2  "a_B"
  Band-Limited White Noise1/1 -> Add1/1
  Bus Selector5/2 -> Derivative/1  "<v_N>"
  Add1/1 -> Bus Creator2/1  "accelerometer_1"
  Bus Selector5/1 -> [r_N]  "<r_N>"
  [r_N] -> Bus Creator2/8
